simulink model "Fan_Control2"  (R2024b)
settings: Solver=FixedStepDiscrete  StartTime=0.0  StopTime=100  FixedStep=1e-4  RelTol=1e-6
values from neighbouring files (symbols this model uses):
  Speed_max = 0.0    [data.sldd]
  Torque_max = 0.0    [data.sldd]
undefined symbols (not defined in the file or in its folder): DiscIntNeverNeededParam
settings Model: DataDictionary=data.sldd  Creator=SESA504213  LastModifiedBy=SESA504213
settings OptimizationCC: ReuseModelBlockBuffer=off  PassReuseOutputArgsAs=Individual arguments  ZeroExternalMemoryAtStartup=off  ZeroInternalMemoryAtStartup=off  OptimizationLevel=level1  OptimizationCustomize=off  EfficientTunableParamExpr=on
settings DebuggingCC: ParameterTunabilityLossMsg=error
settings SFSimCC: MATLABDynamicMemAlloc=off
settings RTWCC: Description=Embedded Coder  SystemTargetFile=ert.tlc  TemplateMakefile=ert_default_tmf  GenerateReport=on  Toolchain=MinGW64 | gmake (64-bit Windows)  BuildConfiguration=Debug  IncludeHyperlinkInReport=on  LaunchReport=on  GenerateTraceInfo=on  GenerateWebview=on  GenerateCodeMetricsReport=on  CheckMdlBeforeBuild=Warning
settings CodeAppCC: ForceParamTrailComments=on  IgnoreCustomStorageClasses=off  OperatorAnnotations=on  SimulinkDataObjDesc=on  SFDataObjDesc=on  CustomSymbolStrBlkIO=$N$M  InsertBlockDesc=on
settings ERTTargetCC: TargetLangStandard=C99 (ISO)  GenerateSampleERTMain=on  CodeInterfacePackaging=Reusable function  InlinedParameterPlacement=Hierarchical  RTWCAPISignals=on  RTWCAPIParams=on  ERTCustomFileTemplate=example_file_process.tlc

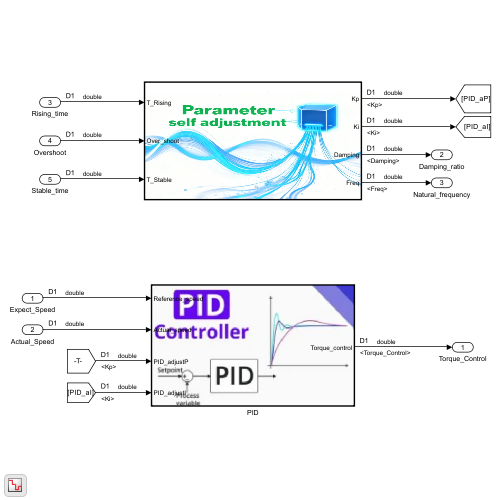
[thumbnail: Simulink's stored preview of the top-level diagram]
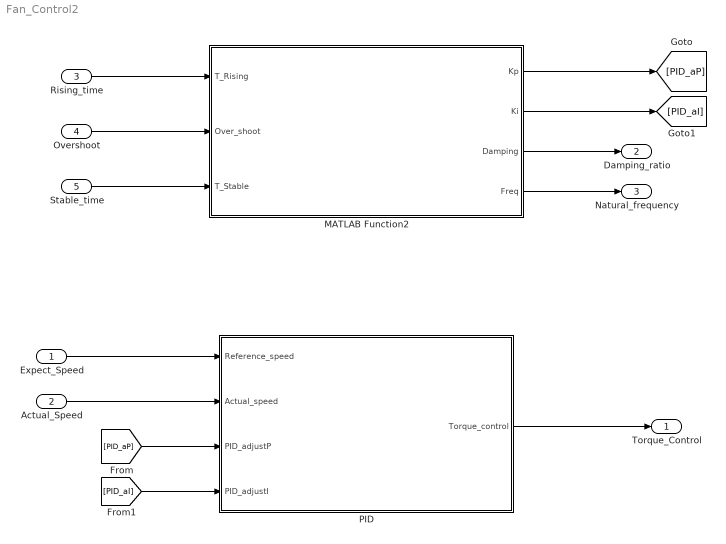
== system Fan_Control2 ==
  Expect_Speed : Inport
  Actual_Speed : Inport  Port=2
  Rising_time : Inport  Port=3
  Overshoot : Inport  Port=4
  Stable_time : Inport  Port=5
  MATLAB Function2 : MATLAB Function  TreatAsAtomicUnit=on  RTWFcnName=PID_Parameter_Adjustment
      settings: RTWFileNameOpts=Use function name
  PID : Subsystem  TreatAsAtomicUnit=on  RTWFcnName=Fan_PID  RTWFileName=Fan_PID
      settings: RTWFcnNameOpts=Use subsystem name  RTWFileNameOpts=Use subsystem name
      mask Display: image('PIDController.jpg');
  Torque_Control : Outport
  Damping_ratio : Outport  Port=2
  Natural_frequency : Outport  Port=3
  wires:
  Expect_Speed/1 -> PID/1(Reference_speed)
  Actual_Speed/1 -> PID/2(Actual_speed)
  PID/1(Torque_control) -> Torque_Control/1
  MATLAB Function2/1(Kp) -> [PID_aP]
  MATLAB Function2/2(Ki) -> [PID_aI]
  [PID_aP] -> PID/3(PID_adjustP)
  [PID_aI] -> PID/4(PID_adjustI)
  Rising_time/1 -> MATLAB Function2/1(T_Rising)
  Overshoot/1 -> MATLAB Function2/2(Over_shoot)
  Stable_time/1 -> MATLAB Function2/3(T_Stable)
  MATLAB Function2/3(Damping) -> Damping_ratio/1
  MATLAB Function2/4(Freq) -> Natural_frequency/1

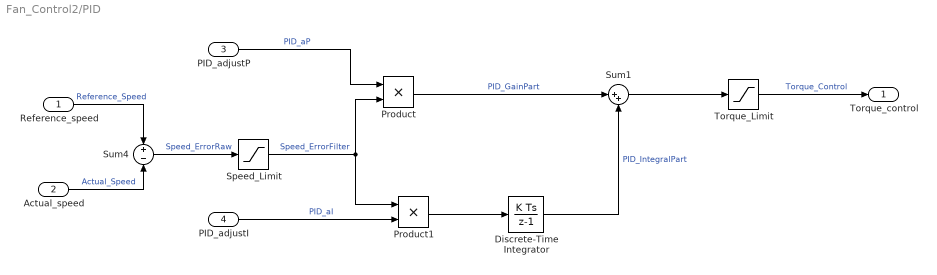
== system Fan_Control2/PID ==
  Reference_speed : Inport
  Actual_speed : Inport  Port=2
  PID_adjustP : Inport  Port=3
  PID_adjustI : Inport  Port=4
  Discrete-Time Integrator : DiscreteIntegrator  SampleTime=-1  LimitOutput=on  UpperSaturationLimit=Torque_max  LowerSaturationLimit=-Torque_max  ICPrevOutput=DiscIntNeverNeededParam  ICPrevScaledInput=DiscIntNeverNeededParam
  Product : Product
  Product1 : Product
  Speed_Limit : Saturate  UpperLimit=Speed_max  LowerLimit=-Speed_max
  Sum1 : Sum  Inputs=|++
  Sum4 : Sum  Inputs=+-
  Torque_Limit : Saturate  UpperLimit=Torque_max  LowerLimit=-Torque_max
  Torque_control : Outport
  wires:
  Product/1 -> Sum1/1  "PID_GainPart"
  Sum1/1 -> Torque_Limit/1
  Torque_Limit/1 -> Torque_control/1  "Torque_Control"
  Reference_speed/1 -> Sum4/1  "Reference_Speed"
  Actual_speed/1 -> Sum4/2  "Actual_Speed"
  Speed_Limit/1 -> Product1/1, Product/2  "Speed_ErrorFilter"
  Sum4/1 -> Speed_Limit/1  "Speed_ErrorRaw"
  PID_adjustP/1 -> Product/1  "PID_aP"
  PID_adjustI/1 -> Product1/2  "PID_aI"
  Product1/1 -> Discrete-Time Integrator/1
  Discrete-Time Integrator/1 -> Sum1/2  "PID_IntegralPart"

== matlab function Fan_Control2/MATLAB Function2 ==
  data: T_Rising input; Kp output; Over_shoot input; T_Stable input; Ki output; Damping output; Freq output
function [Kp, Ki, Damping, Freq] = calc_PI(T_Rising, Over_shoot, T_Stable)
    % Step 1:Calculate the damping ratio zeta from the overshoot M_p 
    Mp_ratio = Over_shoot / 100;   
    if Mp_ratio <= 0 || Mp_ratio >= 1
        error('Overshoot should be in (0,100');
    end
    Damping = -log(Mp_ratio) / sqrt(pi^2 + (log(Mp_ratio))^2);   
    
    % Step 2: Calculate the natural frequency wn from the rise time t_r or settling time t_s (prioritize satisfying t_r)r）
    % t_r ≈ 1.8 / wn（applicable when zeta≈0.7）
    wn_from_tr = 1.8 / T_Rising;
    % t_s（2% error band）：t_s ≈ 4 / (zeta * wn) → wn_from_ts = 4 / (zeta * t_s)
    wn_from_ts = 4 / (Damping * T_Stable);
    
    % Take a more reasonable value from the two（manual adjustment of indicators is required sometimes）
    Freq = (wn_from_tr + wn_from_ts) / 2;  % Compromise 
    
    % Step 3: Derive PI parameters based on the transfer function of the fan's linear model
    % Linear model of the fan：G(s) = 2.857/(s + 0.2334)
    % Closed-loop characteristic equation：s² + (0.2334 + 2.857*Kp)s + 2.857*Ki = s² + 2*zeta*wn*s + wn²
    Kp = (2*Damping*Freq - 0.2334) / 2.857;  % P
    Ki = (Freq^2) / 2.857;                % I
    
    % Ensure parameters are non-negative
    Kp = max(Kp, 0);
    Ki = max(Ki, 0);

    %  Update the model workspace
    %assignin('base', 'PID_P', Kp);
    %assignin('base', 'PID_I', Ki);
end
